simulink model "KP_exemplo"  (R2018b)
settings: Solver=VariableStepAuto  StartTime=0.0  StopTime=50  RelTol=1e-3
values from neighbouring files (symbols this model uses):
  Cd = c2d(C,Ts,'tustin')    [FSP_LINEAR_SISO_exemplo.m]
  F_kp1 = (0.5387*z*(z-0.9457))/(z^2-1.741*z+0.7705)    [FSP_LINEAR_SISO_exemplo.m]
  F_kp2 = (4.9238*z*(z-0.9929)*(z^2-1.93*z+0.9329))/((z-0.9951)*(z-0.7377)*(z^2-1.619*z+0.7105))    [FSP_LINEAR_SISO_exemplo.m]
  Gd = c2d(G,Ts)    [FSP_LINEAR_SISO_exemplo.m]
  Ts = 0.1    [FSP_LINEAR_SISO_exemplo.m]    (also in FSP_NAO_LINEAR_MIMO_cstr.m = 3)
settings Model: Creator=ljffi  LastModifiedBy=ljffi

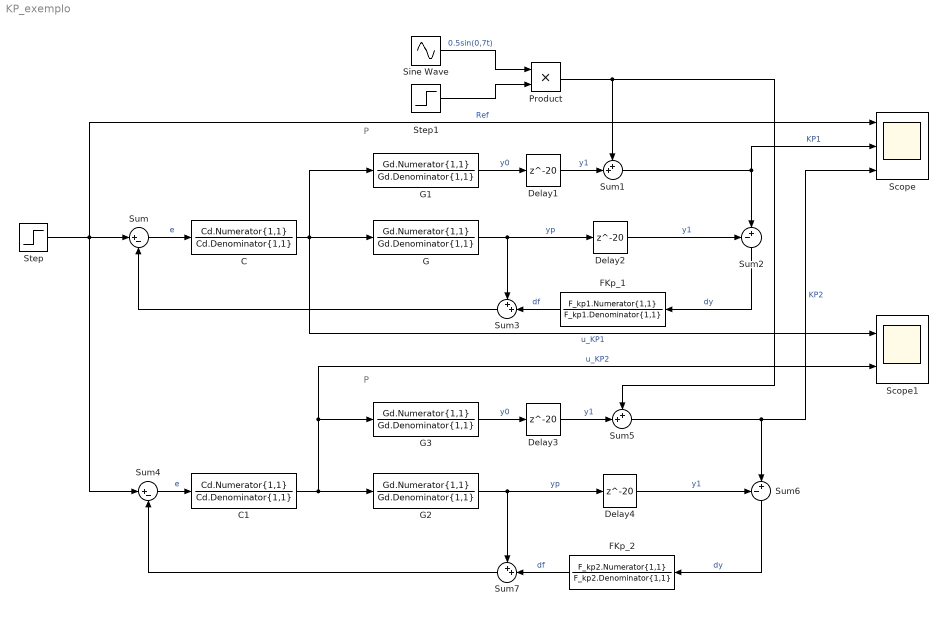
== system KP_exemplo ==
  note: P
  note: P
  C : DiscreteTransferFcn  Numerator=Cd.Numerator{1,1}  Denominator=Cd.Denominator{1,1}  SampleTime=Ts
  C1 : DiscreteTransferFcn  Numerator=Cd.Numerator{1,1}  Denominator=Cd.Denominator{1,1}  SampleTime=Ts
  Delay{1..4} (4 alike) : Delay  DelayLength=20  SampleTime=Ts
  FKp_1 : DiscreteTransferFcn  Numerator=F_kp1.Numerator{1,1}  Denominator=F_kp1.Denominator{1,1}  SampleTime=Ts
  FKp_2 : DiscreteTransferFcn  Numerator=F_kp2.Numerator{1,1}  Denominator=F_kp2.Denominator{1,1}  SampleTime=Ts
  G{,1..3} (4 alike) : DiscreteTransferFcn  Numerator=Gd.Numerator{1,1}  Denominator=Gd.Denominator{1,1}  SampleTime=Ts
  Product : Product
  Scope : Scope  NumInputPorts=3
  Scope1 : Scope  NumInputPorts=2
  Sine Wave : Sin  Amplitude=0.5  Frequency=0.7  Samples=1  SampleTime=Ts
  Step : Step  SampleTime=Ts
  Step1 : Step  Time=20  SampleTime=Ts
  Sum : Sum  Inputs=|+-
  Sum{1,3,5,7} (4 alike) : Sum  Inputs=++|
  Sum2 : Sum  Inputs=-+|
  Sum4 : Sum  Inputs=|+-
  Sum6 : Sum  Inputs=-+|
  wires:
  G/1 -> Delay2/1, Sum3/1  "yp"
  Sum/1 -> C/1  "e"
  Delay2/1 -> Sum2/1  "y1"
  Sum1/1 -> Scope/2, Sum2/2  "KP1"
  Sum2/1 -> FKp_1/1  "dy"
  FKp_1/1 -> Sum3/2  "df"
  Sum3/1 -> Sum/2
  C/1 -> Scope1/1, G1/1, G/1  "u_KP1"
  Step1/1 -> Product/2
  Sine Wave/1 -> Product/1  "0.5sin(0,7t)"
  Delay1/1 -> Sum1/2  "y1"
  G1/1 -> Delay1/1  "y0"
  G3/1 -> Delay3/1  "y0"
  Delay3/1 -> Sum5/2  "y1"
  Product/1 -> Sum5/1, Sum1/1
  Step/1 -> Sum4/1, Scope/1, Sum/1  "Ref"
  C1/1 -> G2/1, Scope1/2, G3/1  "u_KP2"
  Sum7/1 -> Sum4/2
  FKp_2/1 -> Sum7/2  "df"
  Sum6/1 -> FKp_2/1  "dy"
  Sum5/1 -> Scope/3, Sum6/2  "KP2"
  Delay4/1 -> Sum6/1  "y1"
  Sum4/1 -> C1/1  "e"
  G2/1 -> Sum7/1, Delay4/1  "yp"
